simulink model "pmsm"  (R2016a)
settings: Solver=VariableStepAuto  StartTime=0.0  StopTime=1  RelTol=1e-3
libraries: powerlib x21
settings Model: Creator=caijie'  LastModifiedBy=caijie'

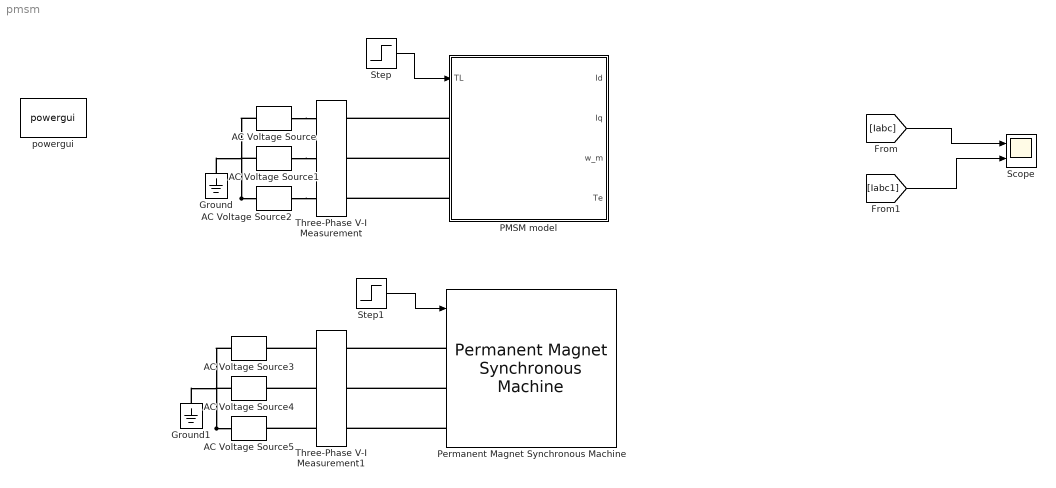
== system pmsm ==
  AC Voltage Source : powerlib/Electrical Sources/AC Voltage Source  Amplitude=220  Phase=0  Frequency=50  SampleTime=0  Measurements=None  BusType=swing  Pref=10e3  Qref=0  Qmin=-inf  Qmax=+inf
  AC Voltage Source1 : powerlib/Electrical Sources/AC Voltage Source  Amplitude=220  Phase=-120  Frequency=50  SampleTime=0  Measurements=None  BusType=swing  Pref=10e3  Qref=0  Qmin=-inf  Qmax=+inf
  AC Voltage Source2 : powerlib/Electrical Sources/AC Voltage Source  Amplitude=220  Phase=120  Frequency=50  SampleTime=0  Measurements=None  BusType=swing  Pref=10e3  Qref=0  Qmin=-inf  Qmax=+inf
  AC Voltage Source3 : powerlib/Electrical Sources/AC Voltage Source  Amplitude=220  Phase=0  Frequency=50  SampleTime=0  Measurements=None  BusType=swing  Pref=10e3  Qref=0  Qmin=-inf  Qmax=+inf
  AC Voltage Source4 : powerlib/Electrical Sources/AC Voltage Source  Amplitude=220  Phase=-120  Frequency=50  SampleTime=0  Measurements=None  BusType=swing  Pref=10e3  Qref=0  Qmin=-inf  Qmax=+inf
  AC Voltage Source5 : powerlib/Electrical Sources/AC Voltage Source  Amplitude=220  Phase=120  Frequency=50  SampleTime=0  Measurements=None  BusType=swing  Pref=10e3  Qref=0  Qmin=-inf  Qmax=+inf
  Ground : powerlib/Elements/Ground  LConnTagsString=a
  Ground1 : powerlib/Elements/Ground  LConnTagsString=a
  "PMSM model " : Subsystem  mask{Ld=8.5e-3, Lq=8.5e-3, Rs=1.3, J=0.0008, p=4, Fai_f=0.175}
      mask prompts: Ld "d轴电感"; Lq "q轴电感"; Rs "电枢电阻"; J "转动惯量"; p "极对数"; Fai_f "磁链"
  Permanent Magnet Synchronous Machine : powerlib/Machines/Permanent Magnet Synchronous Machine  NbPhases=3  FluxDistribution=Sinusoidal  RotorType=Salient-pole  MechanicalLoad=Torque Tm  PresetModel=No  ShowDetailedParameters=on  MeasurementBus=off  Resistance=1.3  Inductance=8.5e-3  dqInductances=[8.5e-3,8.5e-3]  La=0.000835  MachineConstant=Flux linkage established by magnets (V.s)  Flux=0.175  VoltageCst=126.966  TorqueCst=1.05  Flat=120  Mechanical=[0.0008 0 4]  PolePairs=4  InitialConditions=[0,0, 0,0]  InitialConditions5ph=[0 0 0 0 0 0]  TsPowergui=0  TsBlock=-1  RefAngle=Aligned with phase A axis (original Park)
  Scope : Scope  NumInputPorts=2
  Step : Step  Time=0.5  After=50  SampleTime=0
  Step1 : Step  Time=0.5  After=50  SampleTime=0
  Three-Phase V-I Measurement : powerlib/Measurements/Three-Phase V-I Measurement  VoltageMeasurement=phase-to-ground  SetLabelV=on  LabelV=Vabc  Vpu=off  VpuLL=off  CurrentMeasurement=yes  SetLabelI=on  LabelI=Iabc  Ipu=off  Pbase=100e6  Vbase=500e3  OutputType=Complex  PhasorSimulation=off  PSBequivalent=0
  Three-Phase V-I Measurement1 : powerlib/Measurements/Three-Phase V-I Measurement  VoltageMeasurement=phase-to-ground  SetLabelV=on  LabelV=Vabc1  Vpu=off  VpuLL=off  CurrentMeasurement=yes  SetLabelI=on  LabelI=Iabc1  Ipu=off  Pbase=100e6  Vbase=500e3  OutputType=Complex  PhasorSimulation=off  PSBequivalent=0
  powergui : powerlib/powergui  Priority=1  SimulationMode=Discrete  SolverType=Tustin  SampleTime=5e-6  frequency=60  SPID=off  DisableSnubberDevices=off  DisableRonSwitches=off  DisableVfSwitches=off  SwTol=0  DisplayEquations=off  Interpol=off  ExternalGateDelay=off  methode=off  Ts=10  FunctionMessages=off  echomessages=off  HookPort=off  EnableUseOfTLC=off  x0status=blocks  frequencyindice=50  Pbase=100e6  ErrMax=1e-4  Iterations=50  UnitsV=kV  UnitsW=MW  buscounter=0  RestoreLinks=warning  ResistiveCurrentMeasurement=off  Frange=[0:2:500]  Ylog=off  Xlog=on  ShowGrid=off  save=off  variable=ZData  structure=0  ZoomFFT=off  StartTime=0.0  cycles=1  DisplayStyle=1  fundamental=60  FreqAxis=off  MaxFrequency=1000  frequencyindicesteady=1  RmsSteady=1  display=off
  wires:
  Step/1 -> "PMSM model "/1(TL)
  Step1/1 -> Permanent Magnet Synchronous Machine/1
  [Iabc] -> Scope/1
  [Iabc1] -> Scope/2
  connections:
  AC Voltage Source2/LConn1 -- AC Voltage Source/LConn1 -- Ground/LConn1 -- AC Voltage Source1/LConn1
  AC Voltage Source2/RConn1 -- Three-Phase V-I Measurement/LConn3
  AC Voltage Source/RConn1 -- Three-Phase V-I Measurement/LConn1
  "PMSM model "/LConn1 -- Three-Phase V-I Measurement/RConn1
  "PMSM model "/LConn2 -- Three-Phase V-I Measurement/RConn2
  AC Voltage Source1/RConn1 -- Three-Phase V-I Measurement/LConn2
  "PMSM model "/LConn3 -- Three-Phase V-I Measurement/RConn3
  Permanent Magnet Synchronous Machine/LConn1 -- Three-Phase V-I Measurement1/RConn1
  Permanent Magnet Synchronous Machine/LConn2 -- Three-Phase V-I Measurement1/RConn2
  Permanent Magnet Synchronous Machine/LConn3 -- Three-Phase V-I Measurement1/RConn3
  Three-Phase V-I Measurement1/LConn1 -- AC Voltage Source3/RConn1
  AC Voltage Source5/LConn1 -- AC Voltage Source3/LConn1 -- Ground1/LConn1 -- AC Voltage Source4/LConn1
  Three-Phase V-I Measurement1/LConn2 -- AC Voltage Source4/RConn1
  Three-Phase V-I Measurement1/LConn3 -- AC Voltage Source5/RConn1

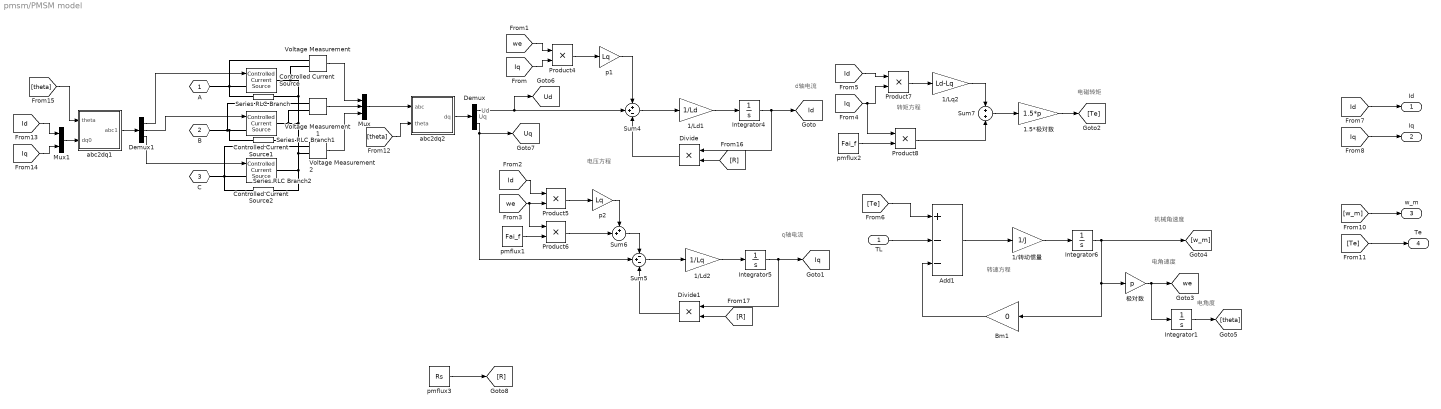
== system pmsm/PMSM model  ==
  note: Uq
  note: Ud
  note: q轴电流
  note: d轴电流
  note: 电磁转矩
  note: 机械角速度
  note: 电角度
  note: 电角速度
  note: 转速方程
  note: 转矩方程
  note: 电压方程
  TL : Inport
  1.5*极对数 : Gain  Gain=1.5*p  SaturateOnIntegerOverflow=on  OutDataTypeStr=Inherit: Same as input  ParamDataTypeStr=Inherit: Same as input
  1/Ld1 : Gain  Gain=1/Ld  SaturateOnIntegerOverflow=on  OutDataTypeStr=Inherit: Same as input  ParamDataTypeStr=Inherit: Same as input
  1/Ld2 : Gain  Gain=1/Lq  SaturateOnIntegerOverflow=on  OutDataTypeStr=Inherit: Same as input  ParamDataTypeStr=Inherit: Same as input
  1/Lq2 : Gain  Gain=Ld-Lq  SaturateOnIntegerOverflow=on  OutDataTypeStr=Inherit: Same as input  ParamDataTypeStr=Inherit: Same as input
  1/转动惯量 : Gain  Gain=1/J  OutDataTypeStr=Inherit: Same as input  ParamDataTypeStr=Inherit: Same as input
  Add1 : Sum  Inputs=+--
  Bm1 : Gain  Gain=0  SaturateOnIntegerOverflow=on  OutDataTypeStr=Inherit: Same as input  ParamDataTypeStr=Inherit: Same as input
  Controlled Current Source : powerlib/Electrical Sources/Controlled Current Source  Initialize=on  Source_Type=AC  Amplitude=0  Phase=0  Frequency=0  Measurements=None
  Controlled Current Source1 : powerlib/Electrical Sources/Controlled Current Source  Initialize=on  Source_Type=AC  Amplitude=0  Phase=0  Frequency=0  Measurements=None
  Controlled Current Source2 : powerlib/Electrical Sources/Controlled Current Source  Initialize=on  Source_Type=AC  Amplitude=0  Phase=0  Frequency=0  Measurements=None
  Demux : Demux  Outputs=2
  Demux1 : Demux  Outputs=3
  Divide : Product  Inputs=**
  Divide1 : Product  Inputs=**
  Integrator{1,4..6} (4 alike) : Integrator
  Mux : Mux  Inputs=3
  Mux1 : Mux  Inputs=2
  Product{4..8} (5 alike) : Product  SaturateOnIntegerOverflow=on  InputSameDT=on  OutDataTypeStr=Inherit: Same as first input
  Series RLC Branch : powerlib/Elements/Series RLC Branch  LConnTagsString=__new0  RConnTagsString=__new0  BranchType=R  Resistance=10000  Inductance=1e-3  SetiL0=off  InitialCurrent=0  Capacitance=1e-6  Setx0=off  InitialVoltage=0  Measurements=None
  Series RLC Branch1 : powerlib/Elements/Series RLC Branch  LConnTagsString=__new0  RConnTagsString=__new0  BranchType=R  Resistance=10000  Inductance=1e-3  SetiL0=off  InitialCurrent=0  Capacitance=1e-6  Setx0=off  InitialVoltage=0  Measurements=None
  Series RLC Branch2 : powerlib/Elements/Series RLC Branch  LConnTagsString=__new0  RConnTagsString=__new0  BranchType=R  Resistance=10000  Inductance=1e-3  SetiL0=off  InitialCurrent=0  Capacitance=1e-6  Setx0=off  InitialVoltage=0  Measurements=None
  Sum4 : Sum  Inputs=++-  SaturateOnIntegerOverflow=on  InputSameDT=on  OutDataTypeStr=Inherit: Same as first input
  Sum5 : Sum  Inputs=-+-  SaturateOnIntegerOverflow=on  InputSameDT=on  OutDataTypeStr=Inherit: Same as first input
  Sum6 : Sum  Inputs=++|  SaturateOnIntegerOverflow=on  InputSameDT=on  OutDataTypeStr=Inherit: Same as first input
  Sum7 : Sum  SaturateOnIntegerOverflow=on  InputSameDT=on  OutDataTypeStr=Inherit: Same as first input
  Voltage Measurement : powerlib/Measurements/Voltage Measurement  PhasorSimulation=off  OutputType=Complex  PSBequivalent=0
  Voltage Measurement1 : powerlib/Measurements/Voltage Measurement  PhasorSimulation=off  OutputType=Complex  PSBequivalent=0
  Voltage Measurement2 : powerlib/Measurements/Voltage Measurement  PhasorSimulation=off  OutputType=Complex  PSBequivalent=0
  abc2dq1 : Subsystem
  abc2dq2 : Subsystem
  p1 : Gain  Gain=Lq  SaturateOnIntegerOverflow=on  OutDataTypeStr=Inherit: Same as input  ParamDataTypeStr=Inherit: Same as input
  p2 : Gain  Gain=Lq  SaturateOnIntegerOverflow=on  OutDataTypeStr=Inherit: Same as input  ParamDataTypeStr=Inherit: Same as input
  pmflux1 : Constant  Value=Fai_f
  pmflux2 : Constant  Value=Fai_f
  pmflux3 : Constant  Value=Rs
  极对数 : Gain  Gain=p  SaturateOnIntegerOverflow=on  OutDataTypeStr=Inherit: Same as input  ParamDataTypeStr=Inherit: Same as input
  A : PMIOPort  Tag=PMCPort  Port=1  Side=Left
  B : PMIOPort  Tag=PMCPort  Port=2  Side=Left
  C : PMIOPort  Tag=PMCPort  Port=3  Side=Left
  Id : Outport
  Iq : Outport  Port=2
  w_m : Outport  Port=3
  Te : Outport  Port=4
  tag scope: Id=global, Iq=global, Ud=global, Uq=global, we=global
  wires:
  Demux/1 -> [Ud], Sum4/2
  Sum4/1 -> 1/Ld1/1
  1/Ld1/1 -> Integrator4/1
  Integrator4/1 -> Divide/1, [Id]
  [we] -> Product4/1
  [Iq] -> Product4/2
  Product4/1 -> p1/1
  p1/1 -> Sum4/1
  Demux/2 -> [Uq], Sum5/2
  Sum5/1 -> 1/Ld2/1
  1/Ld2/1 -> Integrator5/1
  Integrator5/1 -> Divide1/1, [Iq]
  Divide1/1 -> Sum5/3
  [Id] -> Product5/1
  [we] -> Product6/1, Product5/2
  Product5/1 -> p2/1
  Sum6/1 -> Sum5/1
  p2/1 -> Sum6/1
  pmflux1/1 -> Product6/2
  Product6/1 -> Sum6/2
  [Id] -> Product7/1
  [Iq] -> Product8/1, Product7/2
  Product7/1 -> 1/Lq2/1
  pmflux2/1 -> Product8/2
  Product8/1 -> Sum7/2
  1/Lq2/1 -> Sum7/1
  Sum7/1 -> 1.5*极对数/1
  1.5*极对数/1 -> [Te]
  TL/1 -> Add1/2
  [Te] -> Add1/1
  Add1/1 -> 1/转动惯量/1
  1/转动惯量/1 -> Integrator6/1
  Integrator6/1 -> [w_m], 极对数/1, Bm1/1
  Bm1/1 -> Add1/3
  极对数/1 -> Integrator1/1, [we]
  [Id] -> Id/1
  [Iq] -> Iq/1
  Integrator1/1 -> [theta]
  [w_m] -> w_m/1
  [Te] -> Te/1
  Voltage Measurement/1 -> Mux/1
  Voltage Measurement1/1 -> Mux/2
  Voltage Measurement2/1 -> Mux/3
  Mux/1 -> abc2dq2/1(abc)
  [theta] -> abc2dq2/2(theta)
  abc2dq2/1(dq) -> Demux/1
  [Id] -> Mux1/1
  [Iq] -> Mux1/2
  Mux1/1 -> abc2dq1/2(dq0)
  [theta] -> abc2dq1/1(theta)
  abc2dq1/1(abc1) -> Demux1/1
  Demux1/1 -> Controlled Current Source/1
  Demux1/2 -> Controlled Current Source1/1
  Demux1/3 -> Controlled Current Source2/1
  pmflux3/1 -> [R]
  Divide/1 -> Sum4/3
  [R] -> Divide/2
  [R] -> Divide1/2
  connections:
  Series RLC Branch/LConn1 -- Voltage Measurement/LConn1 -- A/RConn1 -- Controlled Current Source/LConn1
  B/RConn1 -- Voltage Measurement1/LConn1 -- Series RLC Branch1/LConn1 -- Controlled Current Source1/LConn1
  C/RConn1 -- Series RLC Branch2/LConn1 -- Voltage Measurement2/LConn1 -- Controlled Current Source2/LConn1
  Controlled Current Source/RConn1 -- Voltage Measurement/LConn2 -- Series RLC Branch/RConn1 -- Series RLC Branch1/RConn1 -- Series RLC Branch2/RConn1 -- Controlled Current Source2/RConn1 -- Voltage Measurement2/LConn2 -- Voltage Measurement1/LConn2 -- Controlled Current Source1/RConn1

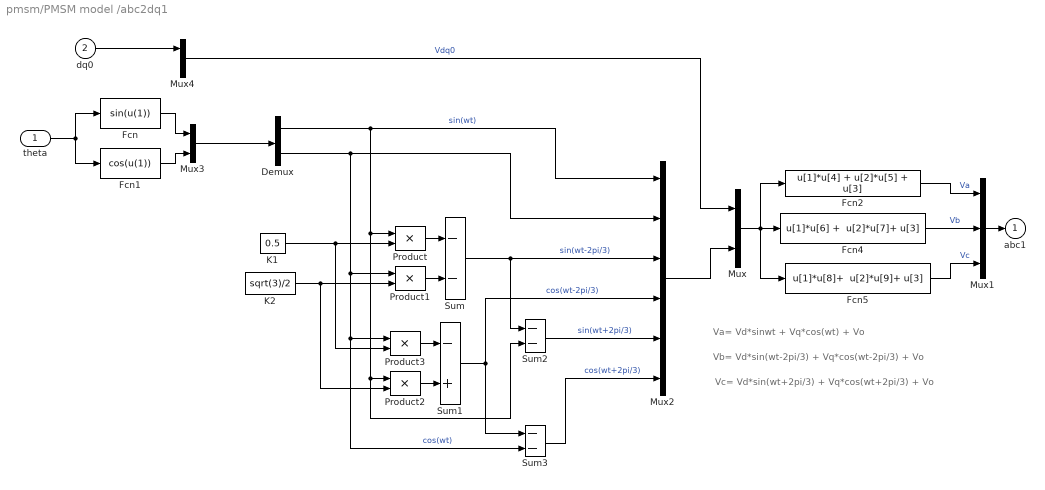
== system pmsm/PMSM model /abc2dq1 ==
  note: Va= Vd*sinwt + Vq*cos(wt) + Vo
  note: Vb= Vd*sin(wt-2pi/3) + Vq*cos(wt-2pi/3) + Vo
  note: Vc= Vd*sin(wt+2pi/3) + Vq*cos(wt+2pi/3) + Vo
  theta : Inport
  dq0 : Inport  Port=2  PortDimensions=2
  Demux : Demux  Outputs=2
  Fcn : Fcn  Expr=sin(u(1))
  Fcn1 : Fcn  Expr=cos(u(1))
  Fcn2 : Fcn  Expr="u[1]*u[4] +  u[2]*u[5] + u[3]"
  Fcn4 : Fcn  Expr="u[1]*u[6] +  u[2]*u[7]+ u[3]"
  Fcn5 : Fcn  Expr="u[1]*u[8]+  u[2]*u[9]+ u[3]"
  K1 : Constant  Value=0.5
  K2 : Constant  Value=sqrt(3)/2
  Mux : Mux  Inputs=2
  Mux1 : Mux  Inputs=3
  Mux2 : Mux  Inputs=6
  Mux3 : Mux  Inputs=2
  Mux4 : Mux  Inputs=2
  Product{,1..3} (4 alike) : Product  SaturateOnIntegerOverflow=on  InputSameDT=on  OutDataTypeStr=Inherit: Same as first input
  Sum : Sum  Inputs=--  SaturateOnIntegerOverflow=on  InputSameDT=on  OutDataTypeStr=Inherit: Same as first input
  Sum1 : Sum  Inputs=-+  SaturateOnIntegerOverflow=on  InputSameDT=on  OutDataTypeStr=Inherit: Same as first input
  Sum2 : Sum  Inputs=--  SaturateOnIntegerOverflow=on  InputSameDT=on  OutDataTypeStr=Inherit: Same as first input
  Sum3 : Sum  Inputs=--  SaturateOnIntegerOverflow=on  InputSameDT=on  OutDataTypeStr=Inherit: Same as first input
  abc1 : Outport  InitialOutput=0
  wires:
  Fcn5/1 -> Mux1/3  "Vc"
  Fcn2/1 -> Mux1/1  "Va"
  Mux1/1 -> abc1/1
  Mux/1 -> Fcn4/1, Fcn2/1, Fcn5/1
  Sum1/1 -> Sum3/1, Mux2/4  "cos(wt-2pi/3)"
  Sum/1 -> Sum2/1, Mux2/3  "sin(wt-2pi/3)"
  K2/1 -> Product2/2, Product1/2
  K1/1 -> Product3/2, Product/2
  Sum2/1 -> Mux2/5  "sin(wt+2pi/3)"
  Sum3/1 -> Mux2/6  "cos(wt+2pi/3)"
  Product2/1 -> Sum1/2
  Product3/1 -> Sum1/1
  Product1/1 -> Sum/2
  Product/1 -> Sum/1
  Demux/1 -> Mux2/1, Sum2/2, Product2/1, Product/1  "sin(wt)"
  Demux/2 -> Mux2/2, Product1/1, Product3/1, Sum3/2  "cos(wt)"
  Mux3/1 -> Demux/1
  Mux2/1 -> Mux/2
  Mux4/1 -> Mux/1  "Vdq0"
  Fcn4/1 -> Mux1/2  "Vb"
  theta/1 -> Fcn1/1, Fcn/1
  Fcn/1 -> Mux3/1
  Fcn1/1 -> Mux3/2
  dq0/1 -> Mux4/1

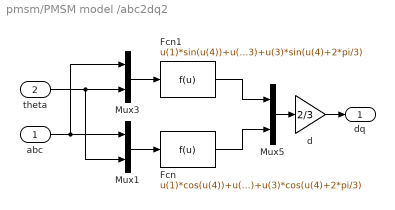
== system pmsm/PMSM model /abc2dq2 ==
  abc : Inport
  theta : Inport  Port=2
  Fcn : Fcn  Expr=u(1)*cos(u(4))+u(2)*cos(u(4)-2*pi/3)+u(3)*cos(u(4)+2*pi/3)
  Fcn1 : Fcn  Expr=u(1)*sin(u(4))+u(2)*sin(u(4)-2*pi/3)+u(3)*sin(u(4)+2*pi/3)
  Mux1 : Mux  Inputs=2
  Mux3 : Mux  Inputs=2
  Mux5 : Mux  Inputs=2
  d : Gain  Gain=2/3  OutDataTypeStr=Inherit: Same as input  ParamDataTypeStr=Inherit: Same as input
  dq : Outport
  wires:
  Mux3/1 -> Fcn1/1
  Fcn1/1 -> Mux5/1
  Mux5/1 -> d/1
  Mux1/1 -> Fcn/1
  Fcn/1 -> Mux5/2
  abc/1 -> Mux1/1, Mux3/1
  theta/1 -> Mux3/2, Mux1/2
  d/1 -> dq/1
